simulink model "zn2_template"  (R2015a)
settings: Solver=ode1  SolverMode=SingleTasking  StartTime=0.0  StopTime=20  FixedStep=0.01  RelTol=1e-3
values from neighbouring files (symbols this model uses):
  KP = 0.6*Ku    (= 6.62800387681)    [exp9.m]    (also in exp9_ptestes.m = 2.42800387681)
  Ku = 4*d/(pi*a)    (= 11.046673128)    [exp9.m]    (also in exp9_ptestes.m = 4.04667312802)
  N = 10    [exp9.m]    (also in exp9_ptestes.m)
  Td = Tu/8    (= 0.0875)    [exp9.m]    (also in exp9_ptestes.m = 0.1275)
  Ti = Tu/2    (= 0.35)    [exp9.m]    (also in exp9_ptestes.m = 0.5)
settings Model: CovSFcnEnable=off  Creator=rpm  LastModifiedBy=Caio
settings DataIOCC: LimitDataPoints=off  SignalLoggingSaveFormat=ModelDataLogs  SaveOutput=off  SignalLogging=off  TimeSaveName=t
settings OptimizationCC: ExpressionDepthLimit=2147483647  InitFltsAndDblsToZero=on
settings DebuggingCC: UnderspecifiedInitializationDetection=Classic  MergeDetectMultiDrivingBlocksExec=none  FcnCallInpInsideContextMsg=UseLocalSettings  StateNameClashWarn=warning
settings GRTTargetCC: CombineOutputUpdateFcns=off  GRTInterface=on

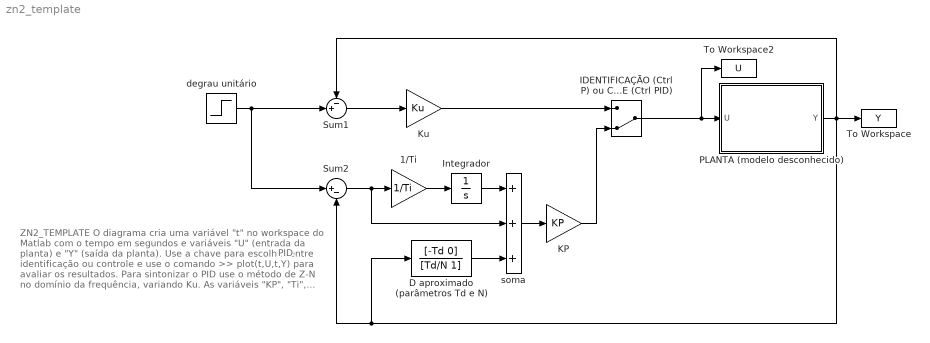
== system zn2_template ==
  note: ZN2_TEMPLATE
      |
      | O diagrama cria uma variável "t" no workspace
      | do Matlab com o tempo em segundos e variáveis
      | "U" (entrada da planta) e "Y" (saída da planta).
      |
      | Use a chave para escolher entre identificação
      | ou controle e use o comando
      |
      | >> plot(t,U,t,Y)
      |
      | para avaliar os resultados.
      |
      | Para sintonizar o PID use o método de Z-N
      | no domínio da frequência, variando Ku.
      |
      | As variáveis "KP", "Ti", "Td" e "N" do Matlab
      | contêm a sintonia do controlador.
      | (é necessário criá-las para que não haja
      | erros na simulação, mesmo se não
      | forem usadas).
      |
      | IMPORTANTE: Não há garantias de que o método
      | seja capaz de produzir um bom desempenho ou
      | mesmo que funcione.
  note: PID
  1/Ti : Gain  Gain=1/Ti
  D aproximado (parâmetros Td e N) : TransferFcn  Numerator=[-Td 0]  Denominator=[Td/N 1]
  IDENTIFICAÇÃO (Ctrl P) ou CONTROLE (Ctrl PID) : ManualSwitch  CurrentSetting=0
  Integrador : Integrator
  KP : Gain  Gain=KP
  Ku : Gain  Gain=Ku
  PLANTA (modelo desconhecido) : Subsystem
  Sum1 : Sum  Inputs=-+|
  Sum2 : Sum  Inputs=|+-
  To Workspace : ToWorkspace  VariableName=Y  SampleTime=-1
  To Workspace2 : ToWorkspace  VariableName=U  SampleTime=-1
  degrau unitário : Step  Time=0  SampleTime=0
  soma : Sum  Inputs=+++
  wires:
  IDENTIFICAÇÃO (Ctrl P) ou CONTROLE (Ctrl PID)/1 -> To Workspace2/1, PLANTA (modelo desconhecido)/1(U)
  degrau unitário/1 -> Sum2/1, Sum1/2
  KP/1 -> IDENTIFICAÇÃO (Ctrl P) ou CONTROLE (Ctrl PID)/2
  soma/1 -> KP/1
  Integrador/1 -> soma/1
  1/Ti/1 -> Integrador/1
  Sum2/1 -> 1/Ti/1, soma/2
  D aproximado (parâmetros Td e N)/1 -> soma/3
  PLANTA (modelo desconhecido)/1(Y) -> To Workspace/1, Sum2/2, D aproximado (parâmetros Td e N)/1, Sum1/1
  Ku/1 -> IDENTIFICAÇÃO (Ctrl P) ou CONTROLE (Ctrl PID)/1
  Sum1/1 -> Ku/1

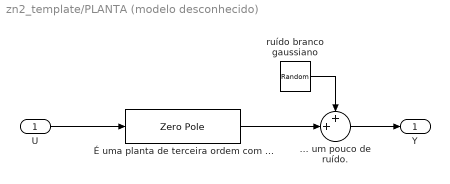
== system zn2_template/PLANTA (modelo desconhecido) ==
  U : Inport
  ... um pouco de ruído. : Sum  Inputs=++|
  ruído branco gaussiano : RandomNumber  Variance=0.001  SampleTime=0
  É uma planta de terceira ordem com ... : ZeroPole  Zeros=[]  Poles=[-1 -2 -3]  Gain=[2]
  Y : Outport
  wires:
  U/1 -> É uma planta de terceira ordem com .../1
  ... um pouco de ruído./1 -> Y/1
  ruído branco gaussiano/1 -> ... um pouco de ruído./1
  É uma planta de terceira ordem com .../1 -> ... um pouco de ruído./2
